simulink model "Sinusoidal_tracking_offset_P3"  (R2022a)
settings: Solver=ode45  StartTime=0.0  StopTime=11  RelTol=1e-3
values from neighbouring files (symbols this model uses):
  A = [0 0 1 0 0 ... (first row only)    [DesignProjectP2.m]    (also in DesignProjectP3.m; DesignProject_OffsetP3.m; mpc_example_regulation.m = [ 	 0,       0,              1,  0, 0; 	 0,       0,        ; mpc_example_tracking.m = [ 	 0,       0,              1,  0, 0; 	 0,       0,        )
  absolute_encoder_counts_per_revolution = 128    [ELEN90064_Project_Parameters.m]
  B = [0;0;0;0;1/La]    [DesignProjectP2.m]    (also in DesignProjectP3.m; DesignProject_OffsetP3.m; mpc_example_regulation.m = [0; 0; 0; 0; 1/La]; mpc_example_tracking.m = [0; 0; 0; 0; 1/La])
  C = [0 1 0 0 0]    [DesignProjectP2.m]    (also in DesignProjectP3.m = [1 0 0 0 0; DesignProject_OffsetP3.m = [1 0 0 0 0; mpc_example_regulation.m = [1 0 0 0 0; mpc_example_tracking.m = [1 0 0 0 0)
  Dp = c2d(Gp, T, 'zoh')    [DesignProjectP3.m]    (also in DesignProject_OffsetP3.m; mpc_example_regulation.m; mpc_example_tracking.m)
  gyro_sigma_drift = deg2rad(5)    [ELEN90064_Project_Parameters.m]
  init = [theta_m_init; theta_l_init; thetadot_m_init; thetadot_l_init; Ia_init]    [ELEN90064_Project_Parameters.m]
  K = K(2:6)    [DesignProjectP2.m]    (also in DesignProjectP3.m = K_dist(1:5); DesignProject_OffsetP3.m = K_dist(2:6); phase2_emc.m = place(A,B,desired_poles))
  K_sin = K_dist(6:7)    [DesignProjectP3.m]    (also in DesignProject_OffsetP3.m = K_dist(7:8))
  Ki = K(1:2)    [DesignProjectP2.m]    (also in DesignProjectP3.m = Kr(1); DesignProject_OffsetP3.m = K_dist(1))
  L_disc = L_disct'    [DesignProjectP3.m]    (also in DesignProject_OffsetP3.m; mpc_example_regulation.m; mpc_example_tracking.m)
  w = 2*pi*1/4    (= 1.57079632679)    [DesignProjectP3.m]    (also in DesignProject_OffsetP3.m)
settings Model: Creator=Admin  LastModifiedBy=Admin
settings DebuggingCC: AlgebraicLoopMsg=none

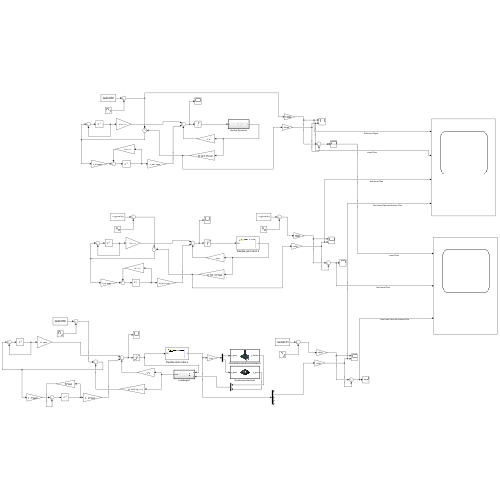
[thumbnail: Simulink's stored preview of the top-level diagram]
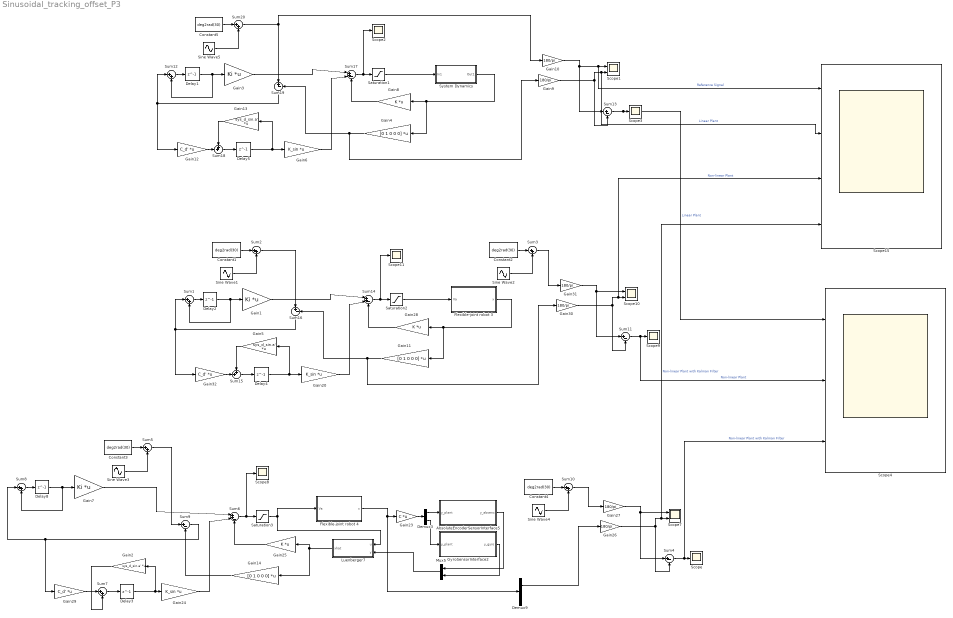
== system Sinusoidal_tracking_offset_P3 ==
  AbsoluteEncoderSensorInterface5 : Subsystem  TreatAsAtomicUnit=on
      mask Display: image('$imagefile'); % Use "Edit Image" on toolstrip to change.
  Constant{1..5} (5 alike) : Constant  Value=deg2rad(30)
  Delay{1..5,8} (6 alike) : Delay  DelayLength=1
  Demux3 : Demux  Outputs=2
  Demux9 : Demux  Outputs=5
  Flexible-joint robot 3 : Subsystem
      mask Display: image('$imagefile'); % Use "Edit Image" on toolstrip to change.
  Flexible-joint robot 4 : Subsystem
      mask Display: image('$imagefile'); % Use "Edit Image" on toolstrip to change.
  Gain1 : Gain  Gain=Ki  Multiplication=Matrix(K*u) (u vector)
  Gain{9..10,26..27,30..31} (6 alike) : Gain  Gain=180/pi
  Gain11 : Gain  Gain=[0 1 0 0 0]  Multiplication=Matrix(K*u) (u vector)
  Gain12 : Gain  Gain=C_d'  Multiplication=Matrix(K*u) (u vector)
  Gain13 : Gain  Gain=sys_d_sin.a'  Multiplication=Matrix(K*u) (u vector)
  Gain14 : Gain  Gain=[0 1 0 0 0]  Multiplication=Matrix(K*u) (u vector)
  Gain2 : Gain  Gain=sys_d_sin.a'  Multiplication=Matrix(K*u) (u vector)
  Gain20 : Gain  Gain=K_sin  Multiplication=Matrix(K*u) (u vector)
  Gain23 : Gain  Gain=C  Multiplication=Matrix(K*u)
  Gain24 : Gain  Gain=K_sin  Multiplication=Matrix(K*u) (u vector)
  Gain25 : Gain  Gain=K  Multiplication=Matrix(K*u)
  Gain28 : Gain  Gain=K  Multiplication=Matrix(K*u)
  Gain29 : Gain  Gain=C_d'  Multiplication=Matrix(K*u) (u vector)
  Gain3 : Gain  Gain=Ki  Multiplication=Matrix(K*u) (u vector)
  Gain32 : Gain  Gain=C_d'  Multiplication=Matrix(K*u) (u vector)
  Gain4 : Gain  Gain=[0 1 0 0 0]  Multiplication=Matrix(K*u) (u vector)
  Gain5 : Gain  Gain=sys_d_sin.a'  Multiplication=Matrix(K*u) (u vector)
  Gain6 : Gain  Gain=K_sin  Multiplication=Matrix(K*u) (u vector)
  Gain7 : Gain  Gain=Ki  Multiplication=Matrix(K*u) (u vector)
  Gain8 : Gain  Gain=K  Multiplication=Matrix(K*u)
  GyroSensorInterface2 : Subsystem  TreatAsAtomicUnit=on
      mask Display: image('$imagefile'); % Use "Edit Image" on toolstrip to change.
  Luenberger7 : Subsystem  TreatAsAtomicUnit=on
  Mux5 : Mux  Inputs=2
  Saturation1 : Saturate  UpperLimit=6  LowerLimit=-6
  Saturation2 : Saturate  UpperLimit=6  LowerLimit=-6
  Saturation3 : Saturate  UpperLimit=6  LowerLimit=-6
  Scope{,2..3,8..9,11} (6 alike) : Scope
  Scope1 : Scope  NumInputPorts=2
  Scope10 : Scope  NumInputPorts=2
  Scope15 : Scope  NumInputPorts=4
  Scope4 : Scope  NumInputPorts=3
  Scope7 : Scope  NumInputPorts=2
  Sine Wave{1..5} (5 alike) : Sin  Amplitude=deg2rad(30)  Frequency=w  Phase=deg2rad(30)  SampleTime=0
  Sum{1..3,5,7..8,10,12,20} (9 alike) : Sum  Inputs=|++
  Sum{4,9,11,13,16,19} (6 alike) : Sum  Inputs=|+-
  Sum14 : Sum  Inputs=|++-
  Sum15 : Sum  Inputs=++|
  Sum17 : Sum  Inputs=|++-
  Sum18 : Sum  Inputs=++|
  Sum6 : Sum  Inputs=|++-
  System Dynamics : Subsystem  TreatAsAtomicUnit=on
  wires:
  Gain11/1 -> Gain30/1, Sum16/2
  Gain30/1 -> Scope15/3, Scope10/2, Sum11/2  "Non-linear Plant"
  Gain5/1 -> Sum15/1
  Delay4/1 -> Gain20/1, Gain5/1
  Flexible-joint robot 3/1(x) -> Gain11/1, Gain28/1
  Sum16/1 -> Sum1/1, Gain32/1
  Gain32/1 -> Sum15/2
  Gain28/1 -> Sum14/3
  Gain31/1 -> Scope10/1, Sum11/1
  Sum2/1 -> Sum16/1
  Sum11/1 -> Scope4/2, Scope9/1  "Non-linear Plant"
  Sum14/1 -> Saturation2/1, Scope11/1
  Gain20/1 -> Sum14/2
  Sum15/1 -> Delay4/1
  Saturation2/1 -> Flexible-joint robot 3/1(Va)
  Delay2/1 -> Gain1/1, Sum1/2
  Sum1/1 -> Delay2/1
  Gain1/1 -> Sum14/1
  Constant1/1 -> Sum2/1
  Sine Wave1/1 -> Sum2/2
  Constant2/1 -> Sum3/1
  Sine Wave2/1 -> Sum3/2
  Sum3/1 -> Gain31/1
  Gain14/1 -> Sum9/2
  Sum4/1 -> Scope4/3, Scope/1  "Non-linear Plant with Kalman Filter"
  Gain23/1 -> Demux3/1
  Demux9/2 -> Gain26/1
  Saturation3/1 -> Flexible-joint robot 4/1(Va), Luenberger7/1(u)
  Mux5/1 -> Luenberger7/2(y)
  Sum5/1 -> Sum9/1
  Gain27/1 -> Scope7/1, Sum4/1
  Flexible-joint robot 4/1(x) -> Demux9/1, Gain23/1
  Gain26/1 -> Scope15/4, Scope7/2, Sum4/2  "Non-linear Plant with Kalman Filter"
  Gain25/1 -> Sum6/3
  Luenberger7/1(xhat) -> Gain14/1, Gain25/1
  Demux3/2 -> GyroSensorInterface2/1(y_plant)
  Sum7/1 -> Delay3/1
  Gain29/1 -> Sum7/1
  Sum6/1 -> Saturation3/1, Scope8/1
  Gain2/1 -> Sum7/2
  Gain24/1 -> Sum6/2
  Delay3/1 -> Gain24/1, Gain2/1
  Demux3/1 -> AbsoluteEncoderSensorInterface5/1(y_plant)
  AbsoluteEncoderSensorInterface5/1(y_absenc) -> Mux5/1
  GyroSensorInterface2/1(y_gyro) -> Mux5/2
  Sum8/1 -> Delay8/1
  Delay8/1 -> Gain7/1, Sum8/2
  Sum9/1 -> Sum8/1, Gain29/1
  Gain7/1 -> Sum6/1
  Constant3/1 -> Sum5/1
  Sine Wave3/1 -> Sum5/2
  Sine Wave4/1 -> Sum10/2
  Constant4/1 -> Sum10/1
  Sum10/1 -> Gain27/1
  Sum20/1 -> Sum19/1, Gain10/1
  Sine Wave5/1 -> Sum20/2
  Constant5/1 -> Sum20/1
  Gain3/1 -> Sum17/1
  Sum12/1 -> Delay1/1
  Delay1/1 -> Sum12/2, Gain3/1
  Saturation1/1 -> System Dynamics/1(In1)
  Sum18/1 -> Delay5/1
  Gain6/1 -> Sum17/2
  Sum17/1 -> Scope2/1, Saturation1/1
  Sum13/1 -> Scope4/1, Scope3/1  "Linear Plant"
  Gain10/1 -> Sum13/1, Scope15/1, Scope1/1  "Reference Signal"
  Gain8/1 -> Sum17/3
  Gain12/1 -> Sum18/2
  Sum19/1 -> Gain12/1, Sum12/1
  System Dynamics/1(Out1) -> Gain8/1, Gain4/1
  Delay5/1 -> Gain13/1, Gain6/1
  Gain13/1 -> Sum18/1
  Gain9/1 -> Sum13/2, Scope15/2, Scope1/2  "Linear Plant"
  Gain4/1 -> Sum19/2, Gain9/1

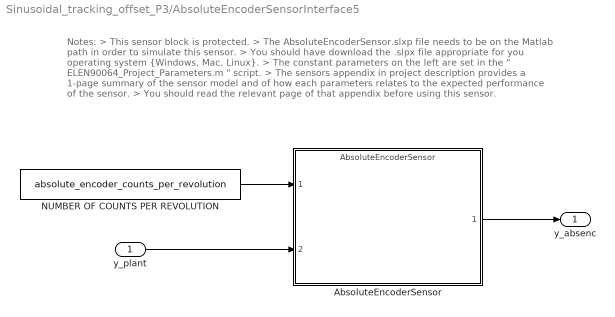
== system Sinusoidal_tracking_offset_P3/AbsoluteEncoderSensorInterface5 ==
  note: Notes:
      | > This sensor block is protected.
      | > The AbsoluteEncoderSensor.slxp file needs to be on the Matlab path in order to simulate this sensor.
      | > You should have download the .slpx file appropriate for you operating system {Windows, Mac, Linux}.
      | > The constant parameters on the left are set in the " ELEN90064_Project_Parameters.m " script.
      | > The sensors appendix in project description provides a 1-page summary of the sensor model and of how each parameters relates to the expected performance of the sensor.
      | > You should read the relevant page of that appendix before using this sensor.
  y_plant : Inport
  AbsoluteEncoderSensor : ModelReference  ModelNameDialog=AbsoluteEncoderSensor.slxp  ModelReferenceVersion=1.16  CopyOfModelProtected=on
  NUMBER OF COUNTS PER REVOLUTION : Constant  Value=absolute_encoder_counts_per_revolution
  y_absenc : Outport
  wires:
  AbsoluteEncoderSensor/1 -> y_absenc/1
  y_plant/1 -> AbsoluteEncoderSensor/2
  NUMBER OF COUNTS PER REVOLUTION/1 -> AbsoluteEncoderSensor/1

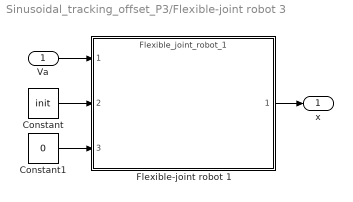
== system Sinusoidal_tracking_offset_P3/Flexible-joint robot 3 ==
  Va : Inport
  Constant : Constant  Value=init
  Constant1 : Constant  Value=0
  Flexible-joint robot 1 : ModelReference  ModelNameDialog=Flexible_joint_robot_1  ModelReferenceVersion=1.65  CopyOfModelProtected=on
  x : Outport
  wires:
  Constant/1 -> Flexible-joint robot 1/2
  Flexible-joint robot 1/1 -> x/1
  Va/1 -> Flexible-joint robot 1/1
  Constant1/1 -> Flexible-joint robot 1/3

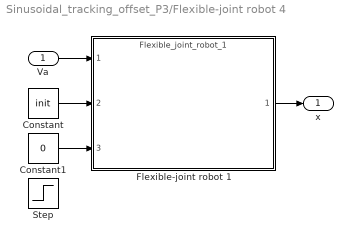
== system Sinusoidal_tracking_offset_P3/Flexible-joint robot 4 ==
  Va : Inport
  Constant : Constant  Value=init
  Constant1 : Constant  Value=0
  Flexible-joint robot 1 : ModelReference  ModelNameDialog=Flexible_joint_robot_1  ModelReferenceVersion=1.65  CopyOfModelProtected=on
  Step : Step  After=0.05  SampleTime=0
  x : Outport
  wires:
  Constant/1 -> Flexible-joint robot 1/2
  Flexible-joint robot 1/1 -> x/1
  Va/1 -> Flexible-joint robot 1/1
  Constant1/1 -> Flexible-joint robot 1/3

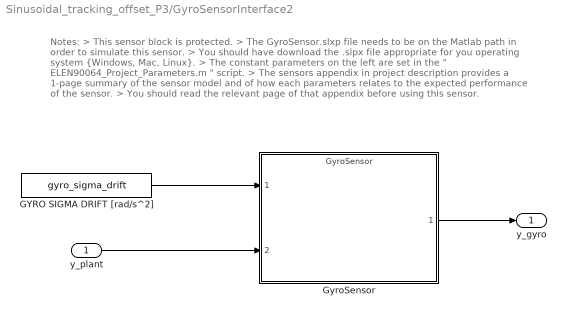
== system Sinusoidal_tracking_offset_P3/GyroSensorInterface2 ==
  note: Notes:
      | > This sensor block is protected.
      | > The GyroSensor.slxp file needs to be on the Matlab path in order to simulate this sensor.
      | > You should have download the .slpx file appropriate for you operating system {Windows, Mac, Linux}.
      | > The constant parameters on the left are set in the " ELEN90064_Project_Parameters.m " script.
      | > The sensors appendix in project description provides a 1-page summary of the sensor model and of how each parameters relates to the expected performance of the sensor.
      | > You should read the relevant page of that appendix before using this sensor.
  y_plant : Inport
  GYRO SIGMA DRIFT [rad/s^2] : Constant  Value=gyro_sigma_drift
  GyroSensor : ModelReference  ModelNameDialog=GyroSensor.slxp  ModelReferenceVersion=1.18  CopyOfModelProtected=on
  y_gyro : Outport
  wires:
  GyroSensor/1 -> y_gyro/1
  y_plant/1 -> GyroSensor/2
  GYRO SIGMA DRIFT [rad/s^2]/1 -> GyroSensor/1

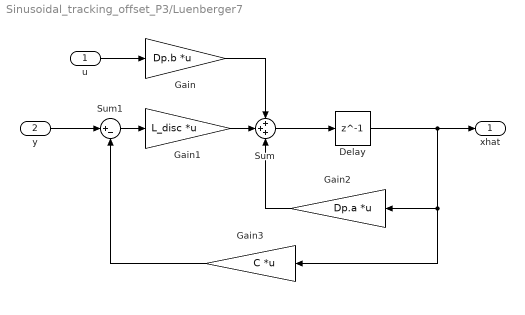
== system Sinusoidal_tracking_offset_P3/Luenberger7 ==
  u : Inport
  y : Inport  Port=2
  Delay : Delay  DelayLength=1
  Gain : Gain  Gain=Dp.b  Multiplication=Matrix(K*u) (u vector)
  Gain1 : Gain  Gain=L_disc  Multiplication=Matrix(K*u) (u vector)
  Gain2 : Gain  Gain=Dp.a  Multiplication=Matrix(K*u) (u vector)
  Gain3 : Gain  Gain=C  Multiplication=Matrix(K*u) (u vector)
  Sum : Sum  Inputs=+++
  Sum1 : Sum  Inputs=|+-
  xhat : Outport
  wires:
  Gain3/1 -> Sum1/2
  Gain2/1 -> Sum/3
  Delay/1 -> xhat/1, Gain2/1, Gain3/1
  Sum/1 -> Delay/1
  Gain1/1 -> Sum/2
  Sum1/1 -> Gain1/1
  y/1 -> Sum1/1
  Gain/1 -> Sum/1
  u/1 -> Gain/1

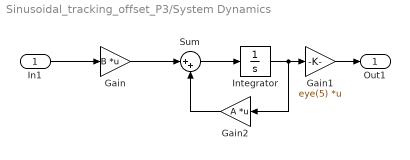
== system Sinusoidal_tracking_offset_P3/System Dynamics ==
  In1 : Inport
  Gain : Gain  Gain=B  Multiplication=Matrix(K*u)
  Gain1 : Gain  Gain=eye(5)  Multiplication=Matrix(K*u)
  Gain2 : Gain  Gain=A  Multiplication=Matrix(K*u)
  Integrator : Integrator
  Sum : Sum  Inputs=|++
  Out1 : Outport
  wires:
  In1/1 -> Gain/1
  Gain/1 -> Sum/1
  Sum/1 -> Integrator/1
  Integrator/1 -> Gain2/1, Gain1/1
  Gain1/1 -> Out1/1
  Gain2/1 -> Sum/2
